simulink model "modello_XY"  (R2021a)
settings: Solver=VariableStepAuto  StartTime=0.0  StopTime=0.2  RelTol=1e-3
undefined symbols (not defined in the file or in its folder): accelerazioni, accelerazioniy, parx, pary
settings Model: Creator=user  LastModifiedBy=stefa
settings SolverCC: AlgebraicLoopSolver=TrustRegion
settings DebuggingCC: SFMachineParentedDataDiag=warning

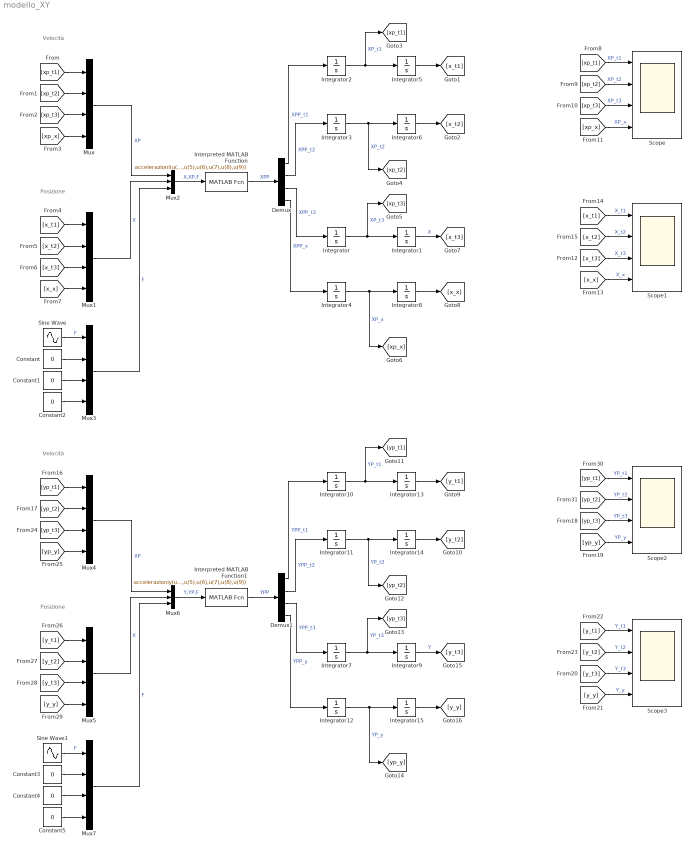
== system modello_XY ==
  note: Posizione
  note: Velocità
  note: Posizione
  note: Velocità
  Constant{,1..5} (6 alike) : Constant  Value=0
  Demux : Demux
  Demux1 : Demux
  Integrator{,2..4,7,10..12} (8 alike) : Integrator
  Integrator1 : Integrator  InitialCondition=parx.V(3,parx.i)
  Integrator13 : Integrator  InitialCondition=pary.Vy(1,pary.i)
  Integrator14 : Integrator  InitialCondition=pary.Vy(2,pary.i)
  Integrator15 : Integrator  InitialCondition=pary.Vy(4,pary.i)
  Integrator5 : Integrator  InitialCondition=parx.V(1,parx.i)
  Integrator6 : Integrator  InitialCondition=parx.V(2,parx.i)
  Integrator8 : Integrator  InitialCondition=parx.V(4,parx.i)
  Integrator9 : Integrator  InitialCondition=pary.Vy(3,pary.i)
  Interpreted MATLAB Function : MATLABFcn  MATLABFcn=accelerazioni(u(1),u(2),u(3),u(4),u(5),u(6),u(7),u(8),u(9))  OutputDimensions=4
  Interpreted MATLAB Function1 : MATLABFcn  MATLABFcn=accelerazioniy(u(1),u(2),u(3),u(4),u(5),u(6),u(7),u(8),u(9))  OutputDimensions=4
  Mux{,1,3..5,7} (6 alike) : Mux
  Mux2 : Mux  Inputs=3
  Mux6 : Mux  Inputs=3
  Scope{,1..3} (4 alike) : Scope  NumInputPorts=4
  Sine Wave : Sin  Amplitude=0  Frequency=600  SampleTime=0
  Sine Wave1 : Sin  Amplitude=0  Frequency=200  SampleTime=0
  wires:
  Interpreted MATLAB Function/1 -> Demux/1  "XPP"
  [xp_t1] -> Mux/1
  [xp_t2] -> Mux/2
  [xp_t3] -> Mux/3
  [xp_x] -> Mux/4
  [x_t3] -> Mux1/3
  [x_t1] -> Mux1/1
  [x_t2] -> Mux1/2
  [x_x] -> Mux1/4
  Mux2/1 -> Interpreted MATLAB Function/1  "X,XP,F"
  Mux/1 -> Mux2/1  "XP"
  Mux1/1 -> Mux2/2  "X"
  [xp_x] -> Scope/4  "XP_x"
  [xp_t3] -> Scope/3  "XP_t3"
  [xp_t2] -> Scope/2  "XP_t2"
  [xp_t1] -> Scope/1  "XP_t1"
  [x_t2] -> Scope1/2  "X_t2"
  [x_t3] -> Scope1/3  "X_t3"
  [x_x] -> Scope1/4  "X_x"
  [x_t1] -> Scope1/1  "X_t1"
  Demux/1 -> Integrator2/1  "XPP_t1"
  Demux/2 -> Integrator3/1  "XPP_t2"
  Demux/3 -> Integrator/1  "XPP_t3"
  Demux/4 -> Integrator4/1  "XPP_x"
  Integrator2/1 -> [xp_t1], Integrator5/1  "XP_t1"
  Integrator3/1 -> [xp_t2], Integrator6/1  "XP_t2"
  Integrator/1 -> [xp_t3], Integrator1/1  "XP_t3"
  Integrator4/1 -> [xp_x], Integrator8/1  "XP_x"
  Integrator5/1 -> [x_t1]
  Integrator6/1 -> [x_t2]
  Integrator1/1 -> [x_t3]  "X"
  Integrator8/1 -> [x_x]
  Sine Wave/1 -> Mux3/1  "F"
  Constant/1 -> Mux3/2
  Constant1/1 -> Mux3/3
  Constant2/1 -> Mux3/4
  Mux3/1 -> Mux2/3  "F"
  Mux6/1 -> Interpreted MATLAB Function1/1  "Y,YP,F"
  Demux1/4 -> Integrator12/1  "YPP_y"
  Integrator12/1 -> [yp_y], Integrator15/1  "YP_y"
  Demux1/3 -> Integrator7/1  "YPP_t3"
  [y_t1] -> Scope3/1  "Y_t1"
  [y_t2] -> Scope3/2  "Y_t2"
  Demux1/1 -> Integrator10/1  "YPP_t1"
  [yp_t3] -> Scope2/3  "YP_t3"
  [y_t3] -> Scope3/3  "Y_t3"
  Demux1/2 -> Integrator11/1  "YPP_t2"
  [yp_y] -> Scope2/4  "YP_y"
  [y_t3] -> Mux5/3
  [yp_t2] -> Mux4/2
  Mux7/1 -> Mux6/3  "F"
  [yp_y] -> Mux4/4
  Interpreted MATLAB Function1/1 -> Demux1/1  "YPP"
  Mux4/1 -> Mux6/1  "XP"
  [yp_t2] -> Scope2/2  "YP_t2"
  [y_y] -> Scope3/4  "Y_y"
  [y_t1] -> Mux5/1
  Constant5/1 -> Mux7/4
  Integrator13/1 -> [y_t1]
  Integrator14/1 -> [y_t2]
  Integrator11/1 -> [yp_t2], Integrator14/1  "YP_t2"
  [yp_t1] -> Mux4/1
  Mux5/1 -> Mux6/2  "X"
  [yp_t3] -> Mux4/3
  Integrator7/1 -> [yp_t3], Integrator9/1  "YP_t3"
  Integrator10/1 -> [yp_t1], Integrator13/1  "YP_t1"
  [yp_t1] -> Scope2/1  "YP_t1"
  Constant3/1 -> Mux7/2
  [y_t2] -> Mux5/2
  Integrator9/1 -> [y_t3]  "Y"
  Sine Wave1/1 -> Mux7/1  "F"
  Integrator15/1 -> [y_y]
  Constant4/1 -> Mux7/3
  [y_y] -> Mux5/4
